simulink model "benchmark_model"  (R2021a)
settings: Solver=ode1  StartTime=0.0  StopTime=Tend  FixedStep=0.0001  MaxStep=0.1  MinStep=0.0001  AbsTol=0.01  EnableMultiTasking=on
undefined symbols (not defined in the file): A1, A2, AL, AM0, AREA, BORE, C_EGR, c_f, c_T, CAIR, cCO, cCO2, cH2, cH2O, cHC, cN2, CO, CO2, cO2, DEN0, DiscIntNeverNeededParam, EGR_dia, EGR_sk, EX_AREA, EX_M_AR, EXO, FD0, FOM, FR0, FR_C1, FR_C2, FR_C3, FR_C4, FR_C5, H2, H2O, HC, INC, INO, KET, Kex, Kh, MAS0, MCh, MHC, MN2, MO2, MOLcylT, N2, O2, PR0, R150, Rabs, SPEC, TBORE, Th_HC, Th_knock, THEX, THIN, TM0 ... (+9)
libraries: pid_lib x1
(part 6 of 6)

== matlab function benchmark_model/ENGINE/engine_s/cylinders/cyl2/cyl/Energy_Int/dvol/func_d_cylvol(u,SPEC)/Embedded MATLAB Function1 ==
  settings: fimath=|
      | fimath(...
      | 'RoundMode', 'floor',...
      | 'OverflowMode', 'wrap',...
      | 'ProductMode', 'KeepLSB', 'ProductWordLength', 32,...
      | 'SumMode', 'KeepLSB', 'SumWordLength', 32,...
      | 'CastBeforeSum', false)
  data: u input; y output; SPEC input size=19
function y = func_d_cylvol(u,SPEC)
%SPEC=[ 1:NCYL;  2:BORE;  3:STROKE;  4:RCRK;  5:CNTL;
%       6:COMP;  7:mc;    8:Jc;      9:cc;   10:mr;
%      11:Jr;   12:cr;   13:mp;     14:cp;   15:a;
%      16:b;    17:y_bdc;18:y_tdc;  19:Jfw;];

BORE   = SPEC(2);
STROKE = SPEC(3);
r      = SPEC(4);
l      = SPEC(5);
COMP   = SPEC(6);

AREA = 0.25*pi*BORE^2;
VH = AREA*STROKE;
VT = VH/(COMP-1);

LL = l^2-(r*sin(u))^2;
y = AREA*r*sin(u)*(1.0+r*cos(u)/sqrt(LL));

== matlab function benchmark_model/ENGINE/engine_s/cylinders/cyl1/ex_valve/cal_flow ==
  data: area input; fen output; inlet input; c_in input; outlet input; c_out input; fml output; WOM input
function [fen,fml] = func_nozzle(area,inlet,c_in,outlet,c_out,WOM) 
% made by Alex on February 3rd, 2010
% This program calculates the flow rate through the nozzle 
% under the assamption that the mass, the energy and the mometum
% are conserved between the inlet and the outlet flows.
%
% The inlet and the outlet are connected with the sign convention 
% of the calculated flow. The sign of the flow from th einlet and 
% the outlet is positive.
%
% inlet(1):pressure 
% inlet(2):density
% inlet(3):weight of molecule
% inlet(4):degree of freedom
% outlet(1):pressure 
% outlet(2):density
% outlet(3):weight of molecule
% outlet(4):degree of freedom

y = zeros(8,1); % modified 

du = inlet(1);
pu = inlet(2);
mu = inlet(3);
fu = inlet(4);
dd = outlet(1);
if dd<0
    dd=0;
end
pd = outlet(2);
md = outlet(3);
fd = outlet(4);
AR = area;

if (pu >= pd)
    rp = pd/pu;
    k = (fu + 2.0)/fu;
    crp = 1.0/(k + 1.0);
    A = AR*sqrt((k + 1.0)/(2.0*k)*abs(pu*du));
    B = sqrt((k/(k + 1.0))^2 - (0.99 - 1.0/(k + 1.0))^2);
    C = -(0.99 - 1.0/(k + 1.0))/B;
    a = (C*0.01 - B)/(2.0*0.01^3);
    c = C - 3.0*a*0.01^2;
    if (rp >= 0.99)
      fms = A*(a*(1.0 - rp)^3 + c*(1.0 - rp));
    else
      if (rp >= crp)
        R = (k/(k + 1.0))^2 - (rp - 1.0/(k + 1.0))^2;
        if (R < 0)
          R = 0;
        end
        fms = A*sqrt(R);
      else
        fms = A*k/(k + 1.0);
      end
    end
    fen = fms*(fu + 2.0)/2.0*pu/du;
    Ma = WOM'*c_in;
    fml = c_in*fms/Ma;
  else
    rp = pu/pd;
    k = (fd + 2.0)/fd;
    crp = 1.0/(k + 1.0);
    A = AR*sqrt((k + 1.0)/(2.0*k)*pd*dd);
    B = sqrt((k/(k + 1.0))^2 - (0.99 - 1.0/(k + 1.0))^2);
    C = (0.99 - 1.0/(k + 1.0))/B;
    a = (C*0.01 - B)/(2.0*0.01^3);
    c = C - 3.0*a*0.01^2;
    if (rp >= 0.99)
      fms = -A*(a*(1.0 - rp)^3 + c*(1.0 - rp));
    else
      if (rp >= crp)
        R = (k/(k + 1.0))^2 - (rp - 1.0/(k + 1.0))^2;
        if (R < 0)
          R = 0;
        end
        fms = -A*sqrt(R);
      else
        fms = -A*k/(k + 1.0);
      end
    end
    fen = fms*(fd + 2.0)/2.0*pd/dd;
    if isnan(fen)
        fen=0;
    end

    Ma = WOM'*c_out;
    fml = c_out*fms/Ma;
end
 if isnan(fen)||isinf(fen)
       fen=0;
end

== matlab function benchmark_model/ENGINE/engine_s/cylinders/cyl4/ex_valve/cal_flow ==
  data: area input; fen output; inlet input; c_in input; outlet input; c_out input; fml output; WOM input
function [fen,fml] = func_nozzle(area,inlet,c_in,outlet,c_out,WOM) 
% made by Alex on February 3rd, 2010
% This program calculates the flow rate through the nozzle 
% under the assamption that the mass, the energy and the mometum
% are conserved between the inlet and the outlet flows.
%
% The inlet and the outlet are connected with the sign convention 
% of the calculated flow. The sign of the flow from th einlet and 
% the outlet is positive.
%
% inlet(1):pressure 
% inlet(2):density
% inlet(3):weight of molecule
% inlet(4):degree of freedom
% outlet(1):pressure 
% outlet(2):density
% outlet(3):weight of molecule
% outlet(4):degree of freedom

y = zeros(8,1); % modified 

du = inlet(1);
pu = inlet(2);
mu = inlet(3);
fu = inlet(4);
dd = outlet(1);
if dd<0
    dd=0;
end
pd = outlet(2);
md = outlet(3);
fd = outlet(4);
AR = area;

if (pu >= pd)
    rp = pd/pu;
    k = (fu + 2.0)/fu;
    crp = 1.0/(k + 1.0);
    A = AR*sqrt((k + 1.0)/(2.0*k)*pu*du);
    B = sqrt((k/(k + 1.0))^2 - (0.99 - 1.0/(k + 1.0))^2);
    C = -(0.99 - 1.0/(k + 1.0))/B;
    a = (C*0.01 - B)/(2.0*0.01^3);
    c = C - 3.0*a*0.01^2;
    if (rp >= 0.99)
      fms = A*(a*(1.0 - rp)^3 + c*(1.0 - rp));
    else
      if (rp >= crp)
        R = (k/(k + 1.0))^2 - (rp - 1.0/(k + 1.0))^2;
        if (R < 0)
          R = 0;
        end
        fms = A*sqrt(R);
      else
        fms = A*k/(k + 1.0);
      end
    end
    fen = fms*(fu + 2.0)/2.0*pu/du;
    Ma = WOM'*c_in;
    fml = c_in*fms/Ma;
  else
    rp = pu/pd;
    k = (fd + 2.0)/fd;
    crp = 1.0/(k + 1.0);
    A = AR*sqrt((k + 1.0)/(2.0*k)*pd*dd);
    B = sqrt((k/(k + 1.0))^2 - (0.99 - 1.0/(k + 1.0))^2);
    C = (0.99 - 1.0/(k + 1.0))/B;
    a = (C*0.01 - B)/(2.0*0.01^3);
    c = C - 3.0*a*0.01^2;
    if (rp >= 0.99)
      fms = -A*(a*(1.0 - rp)^3 + c*(1.0 - rp));
    else
      if (rp >= crp)
        R = (k/(k + 1.0))^2 - (rp - 1.0/(k + 1.0))^2;
        if (R < 0)
          R = 0;
        end
        fms = -A*sqrt(R);
      else
        fms = -A*k/(k + 1.0);
      end
    end
    fen = fms*(fd + 2.0)/2.0*pd/dd;
    Ma = WOM'*c_out;
    fml = c_out*fms/Ma;
end
if isnan(fen)
       fen=0;
end

== matlab function benchmark_model/ENGINE/engine_s/cylinders/cyl4/in_valve/cal_flow ==
  data: area input; fen output; inlet input; c_in input; outlet input; c_out input; fml output; fms output; WOM input
function [fen,fml,fms] = func_nozzle(area,inlet,c_in,outlet,c_out,WOM) 
% made by Alex on February 3rd, 2010
% This program calculates the flow rate through the nozzle 
% under the assamption that the mass, the energy and the mometum
% are conserved between the inlet and the outlet flows.
%
% The inlet and the outlet are connected with the sign convention 
% of the calculated flow. The sign of the flow from th einlet and 
% the outlet is positive.
%
% inlet(1):pressure 
% inlet(2):density
% inlet(3):weight of molecule
% inlet(4):degree of freedom
% outlet(1):pressure 
% outlet(2):density
% outlet(3):weight of molecule
% outlet(4):degree of freedom

y = zeros(8,1); % modified 

du = inlet(1);
pu = inlet(2);
mu = inlet(3);
fu = inlet(4);
dd = outlet(1);
pd = outlet(2);
md = outlet(3);
fd = outlet(4);
AR = area;

if (pu >= pd)
    rp = pd/pu;
    k = (fu + 2.0)/fu;
    crp = 1.0/(k + 1.0);
    A = AR*sqrt((k + 1.0)/(2.0*k)*pu*du);
    B = sqrt((k/(k + 1.0))^2 - (0.99 - 1.0/(k + 1.0))^2);
    C = -(0.99 - 1.0/(k + 1.0))/B;
    a = (C*0.01 - B)/(2.0*0.01^3);
    c = C - 3.0*a*0.01^2;
    if (rp >= 0.99)
      fms = A*(a*(1.0 - rp)^3 + c*(1.0 - rp));
    else
      if (rp >= crp)
        R = (k/(k + 1.0))^2 - (rp - 1.0/(k + 1.0))^2;
        if (R < 0)
          R = 0;
        end
        fms = A*sqrt(R);
      else
        fms = A*k/(k + 1.0);
      end
    end
    fen = fms*(fu + 2.0)/2.0*pu/du;
    Ma = WOM'*c_in;
    fml = c_in*fms/Ma;
  else
    rp = pu/pd;
    k = (fd + 2.0)/fd;
    crp = 1.0/(k + 1.0);
    A = AR*sqrt((k + 1.0)/(2.0*k)*pd*dd);
    B = sqrt((k/(k + 1.0))^2 - (0.99 - 1.0/(k + 1.0))^2);
    C = (0.99 - 1.0/(k + 1.0))/B;
    a = (C*0.01 - B)/(2.0*0.01^3);
    c = C - 3.0*a*0.01^2;
    if (rp >= 0.99)
      fms = -A*(a*(1.0 - rp)^3 + c*(1.0 - rp));
    else
      if (rp >= crp)
        R = (k/(k + 1.0))^2 - (rp - 1.0/(k + 1.0))^2;
        if (R < 0)
          R = 0;
        end
        fms = -A*sqrt(R);
      else
        fms = -A*k/(k + 1.0);
      end
    end
    fen = fms*(fd + 2.0)/2.0*pd/dd;
    Ma = WOM'*c_out;
    fml = c_out*fms/Ma;
end
if isnan(fen)
    fen=0;
end

== matlab function benchmark_model/ENGINE/engine_s/cylinders/cyl1/in_valve/cal_flow ==
  data: area input; fen output; inlet input; c_in input; outlet input; c_out input; fml output; fms output; WOM input
function [fen,fml,fms] = func_nozzle(area,inlet,c_in,outlet,c_out,WOM) 
% made by Alex on February 3rd, 2010
% This program calculates the flow rate through the nozzle 
% under the assamption that the mass, the energy and the mometum
% are conserved between the inlet and the outlet flows.
%
% The inlet and the outlet are connected with the sign convention 
% of the calculated flow. The sign of the flow from th einlet and 
% the outlet is positive.
%
% inlet(1):pressure 
% inlet(2):density
% inlet(3):weight of molecule
% inlet(4):degree of freedom
% outlet(1):pressure 
% outlet(2):density
% outlet(3):weight of molecule
% outlet(4):degree of freedom

y = zeros(8,1); % modified 

du = inlet(1);
pu = inlet(2);
mu = inlet(3);
fu = inlet(4);
dd = outlet(1);
if dd<0
    dd=0;
end
pd = outlet(2);
md = outlet(3);
fd = outlet(4);
AR = area;

if (pu >= pd)
    rp = pd/pu;
    k = (fu + 2.0)/fu;
    crp = 1.0/(k + 1.0);
    A = AR*sqrt((k + 1.0)/(2.0*k)*pu*du);
    B = sqrt((k/(k + 1.0))^2 - (0.99 - 1.0/(k + 1.0))^2);
    C = -(0.99 - 1.0/(k + 1.0))/B;
    a = (C*0.01 - B)/(2.0*0.01^3);
    c = C - 3.0*a*0.01^2;
    if (rp >= 0.99)
      fms = A*(a*(1.0 - rp)^3 + c*(1.0 - rp));
    else
      if (rp >= crp)
        R = (k/(k + 1.0))^2 - (rp - 1.0/(k + 1.0))^2;
        if (R < 0)
          R = 0;
        end
        fms = A*sqrt(R);
      else
        fms = A*k/(k + 1.0);
      end
    end
    fen = fms*(fu + 2.0)/2.0*pu/du;
    Ma = WOM'*c_in;
    fml = c_in*fms/Ma;
  else
    rp = pu/pd;
    k = (fd + 2.0)/fd;
    crp = 1.0/(k + 1.0);
    A = AR*sqrt((k + 1.0)/(2.0*k)*pd*dd);
    B = sqrt((k/(k + 1.0))^2 - (0.99 - 1.0/(k + 1.0))^2);
    C = (0.99 - 1.0/(k + 1.0))/B;
    a = (C*0.01 - B)/(2.0*0.01^3);
    c = C - 3.0*a*0.01^2;
    if (rp >= 0.99)
      fms = -A*(a*(1.0 - rp)^3 + c*(1.0 - rp));
    else
      if (rp >= crp)
        R = (k/(k + 1.0))^2 - (rp - 1.0/(k + 1.0))^2;
        if (R < 0)
          R = 0;
        end
        fms = -A*sqrt(R);
      else
        fms = -A*k/(k + 1.0);
      end
    end
    fen = fms*(fd + 2.0)/2.0*pd/dd;
    Ma = WOM'*c_out;
    fml = c_out*fms/Ma;
end
if isnan(fen)
       fen=0;
end

== matlab function benchmark_model/ENGINE/engine_s/in_chamber/cal_flow ==
  data: area input; fen output; inlet input; c_in input; outlet input; c_out input; fml output; WOM input
function [fen,fml] = func_nozzle(area,inlet,c_in,outlet,c_out,WOM) 
% made by Alex on February 3rd, 2010
% This program calculates the flow rate through the nozzle 
% under the assamption that the mass, the energy and the mometum
% are conserved between the inlet and the outlet flows.
%
% The inlet and the outlet are connected with the sign convention 
% of the calculated flow. The sign of the flow from th einlet and 
% the outlet is positive.
%
% inlet(1):pressure 
% inlet(2):density
% inlet(3):weight of molecule
% inlet(4):degree of freedom
% outlet(1):pressure 
% outlet(2):density
% outlet(3):weight of molecule
% outlet(4):degree of freedom

y = zeros(8,1); % modified 

du = inlet(1);
pu = inlet(2);
mu = inlet(3);
fu = inlet(4);
dd = outlet(1);
pd = outlet(2);
md = outlet(3);
fd = outlet(4);
AR = area;

if (pu >= pd)
    rp = pd/pu;
    k = (fu + 2.0)/fu;
    crp = 1.0/(k + 1.0);
    A = AR*sqrt((k + 1.0)/(2.0*k)*pu*du);
    B = sqrt((k/(k + 1.0))^2 - (0.99 - 1.0/(k + 1.0))^2);
    C = -(0.99 - 1.0/(k + 1.0))/B;
    a = (C*0.01 - B)/(2.0*0.01^3);
    c = C - 3.0*a*0.01^2;
    if (rp >= 0.99)
      fms = A*(a*(1.0 - rp)^3 + c*(1.0 - rp));
    else
      if (rp >= crp)
        R = (k/(k + 1.0))^2 - (rp - 1.0/(k + 1.0))^2;
        if (R < 0)
          R = 0;
        end
        fms = A*sqrt(R);
      else
        fms = A*k/(k + 1.0);
      end
    end
    fen = fms*(fu + 2.0)/2.0*pu/du;
    Ma = WOM'*c_in;
    fml = c_in*fms/Ma;
  else
    rp = pu/pd;
    k = (fd + 2.0)/fd;
    crp = 1.0/(k + 1.0);
    A = AR*sqrt((k + 1.0)/(2.0*k)*pd*dd);
    B = sqrt((k/(k + 1.0))^2 - (0.99 - 1.0/(k + 1.0))^2);
    C = (0.99 - 1.0/(k + 1.0))/B;
    a = (C*0.01 - B)/(2.0*0.01^3);
    c = C - 3.0*a*0.01^2;
    if (rp >= 0.99)
      fms = -A*(a*(1.0 - rp)^3 + c*(1.0 - rp));
    else
      if (rp >= crp)
        R = (k/(k + 1.0))^2 - (rp - 1.0/(k + 1.0))^2;
        if (R < 0)
          R = 0;
        end
        fms = -A*sqrt(R);
      else
        fms = -A*k/(k + 1.0);
      end
    end
    fen = fms*(fd + 2.0)/2.0*pd/dd;
    Ma = WOM'*c_out;
    fml = c_out*fms/Ma;
end

== matlab function benchmark_model/ENGINE/engine_s/EGR_system/cal_flow ==
  data: area input; fen output; inlet input; c_in input; outlet input; c_out input; fml output; WOM input
function [fen,fml] = func_nozzle(area,inlet,c_in,outlet,c_out,WOM) 
% made by Alex on February 3rd, 2010
% This program calculates the flow rate through the nozzle 
% under the assamption that the mass, the energy and the mometum
% are conserved between the inlet and the outlet flows.
%
% The inlet and the outlet are connected with the sign convention 
% of the calculated flow. The sign of the flow from th einlet and 
% the outlet is positive.
%
% inlet(1):pressure 
% inlet(2):density
% inlet(3):weight of molecule
% inlet(4):degree of freedom
% outlet(1):pressure 
% outlet(2):density
% outlet(3):weight of molecule
% outlet(4):degree of freedom

y = zeros(8,1); % modified 
du = inlet(1);
if du<0
    du=0;
end
pu = inlet(2);
mu = inlet(3);
fu = inlet(4);
dd = outlet(1);
pd = outlet(2);
md = outlet(3);
fd = outlet(4);
AR = area;

if (pu >= pd)
    rp = pd/pu;
    k = (fu + 2.0)/fu;
    crp = 1.0/(k + 1.0);
    A = AR*sqrt((k + 1.0)/(2.0*k)*pu*du);
    B = sqrt((k/(k + 1.0))^2 - (0.99 - 1.0/(k + 1.0))^2);
    C = -(0.99 - 1.0/(k + 1.0))/B;
    a = (C*0.01 - B)/(2.0*0.01^3);
    c = C - 3.0*a*0.01^2;
    if (rp >= 0.99)
      fms = A*(a*(1.0 - rp)^3 + c*(1.0 - rp));
    else
      if (rp >= crp)
        R = (k/(k + 1.0))^2 - (rp - 1.0/(k + 1.0))^2;
        if (R < 0)
          R = 0;
        end
        fms = A*sqrt(R);
      else
        fms = A*k/(k + 1.0);
      end
    end
    fen = fms*(fu + 2.0)/2.0*pu/du;
    Ma = WOM'*c_in;
    fml = c_in*fms/Ma;
  else
    rp = pu/pd;
    k = (fd + 2.0)/fd;
    crp = 1.0/(k + 1.0);
    A = AR*sqrt((k + 1.0)/(2.0*k)*pd*dd);
    B = sqrt((k/(k + 1.0))^2 - (0.99 - 1.0/(k + 1.0))^2);
    C = (0.99 - 1.0/(k + 1.0))/B;
    a = (C*0.01 - B)/(2.0*0.01^3);
    c = C - 3.0*a*0.01^2;
    if (rp >= 0.99)
      fms = -A*(a*(1.0 - rp)^3 + c*(1.0 - rp));
    else
      if (rp >= crp)
        R = (k/(k + 1.0))^2 - (rp - 1.0/(k + 1.0))^2;
        if (R < 0)
          R = 0;
        end
        fms = -A*sqrt(R);
      else
        fms = -A*k/(k + 1.0);
      end
    end
    fen = fms*(fd + 2.0)/2.0*pd/dd;
    Ma = WOM'*c_out;
    fml = c_out*fms/Ma;
end
if isnan(fen)
       fen=0;
end

== matlab function benchmark_model/ENGINE/engine_s/cylinders/cyl2/cyl/cal_cyl_state/cyl_vol ==
  settings: fimath=|
      | fimath(...
      | 'RoundMode', 'floor',...
      | 'OverflowMode', 'wrap',...
      | 'ProductMode', 'KeepLSB', 'ProductWordLength', 32,...
      | 'SumMode', 'KeepLSB', 'SumWordLength', 32,...
      | 'CastBeforeSum', false)
  data: u input; vol output; SPEC input size=19
function vol=func_cylvol(u,SPEC)
%SPEC=[ 1:NCYL;  2:BORE;  3:STROKE;  4:RCRK;  5:CNTL;
%       6:COMP;  7:mc;    8:Jc;      9:cc;   10:mr;
%      11:Jr;   12:cr;   13:mp;     14:cp;   15:a;
%      16:b;    17:y_bdc;18:y_tdc;  19:Jfw;];

   r    = SPEC(4);
   l    = SPEC(5);
   
   AREA = 0.25*pi*SPEC(2)*SPEC(2);
   VH = AREA*SPEC(3);
   VT = VH/(SPEC(6)-1);
   LL = l^2-(r*sin(u))^2;
   vol = VT+AREA*((r+l)-(r*cos(u)+sqrt(LL)));

== matlab function benchmark_model/ENGINE/engine_s/cylinders/cyl2/cyl/frame/ratio_burnt1/murnt_ratio/Embedded MATLAB Function ==
  data: u input; q output; Web input; Q output
function [q,Q]  = func_webC_s(u,Web)
% made by Alex on January 28th, 2010
%   y: burnt ratio
%   u: crank angle that takes 0 at the compression TDC
% Web: parameters
%
WebA = Web(1);
WebM = Web(2);
WebT = Web(3);
WebS = Web(4);
WWebs = pi-WebS;

uu = mod(u,4*pi)-WWebs;
if (uu>0)   
    q = 1.0/WebT*(WebM+1.0)*WebA*(uu/WebT)^WebM*...
          exp(-WebA*(uu/WebT)^(WebM+1.0));
    Q = 1-exp(-WebA*(uu/WebT)^(WebM+1.0));
else
    q = 0;
    Q = 0;
end

== matlab function benchmark_model/ENGINE/engine_s/ex_chamber/cal_flow ==
  data: area input; fen output; inlet input; c_in input; outlet input; c_out input; fml output; WOM input
function [fen,fml] = func_nozzle(area,inlet,c_in,outlet,c_out,WOM) 
% made by Alex on February 3rd, 2010
% This program calculates the flow rate through the nozzle 
% under the assamption that the mass, the energy and the mometum
% are conserved between the inlet and the outlet flows.
%
% The inlet and the outlet are connected with the sign convention 
% of the calculated flow. The sign of the flow from th einlet and 
% the outlet is positive.
%
% inlet(1):pressure 
% inlet(2):density
% inlet(3):weight of molecule
% inlet(4):degree of freedom
% outlet(1):pressure 
% outlet(2):density
% outlet(3):weight of molecule
% outlet(4):degree of freedom

y = zeros(8,1); % modified 

du = inlet(1);
if du<0
    du=0;
end
pu = inlet(2);
mu = inlet(3);
fu = inlet(4);
dd = outlet(1);
pd = outlet(2);
md = outlet(3);
fd = outlet(4);
AR = area;

if (pu >= pd)
    rp = pd/pu;
    k = (fu + 2.0)/fu;
    crp = 1.0/(k + 1.0);
    A = AR*sqrt((k + 1.0)/(2.0*k)*pu*du);
    B = sqrt((k/(k + 1.0))^2 - (0.99 - 1.0/(k + 1.0))^2);
    C = -(0.99 - 1.0/(k + 1.0))/B;
    a = (C*0.01 - B)/(2.0*0.01^3);
    c = C - 3.0*a*0.01^2;
    if (rp >= 0.99)
      fms = A*(a*(1.0 - rp)^3 + c*(1.0 - rp));
    else
      if (rp >= crp)
        R = (k/(k + 1.0))^2 - (rp - 1.0/(k + 1.0))^2;
        if (R < 0)
          R = 0;
        end
        fms = A*sqrt(R);
      else
        fms = A*k/(k + 1.0);
      end
    end
    fen = fms*(fu + 2.0)/2.0*pu/du;
    Ma = WOM'*c_in;
    fml = c_in*fms/Ma;
  else
    rp = pu/pd;
    k = (fd + 2.0)/fd;
    crp = 1.0/(k + 1.0);
    A = AR*sqrt((k + 1.0)/(2.0*k)*pd*dd);
    B = sqrt((k/(k + 1.0))^2 - (0.99 - 1.0/(k + 1.0))^2);
    C = (0.99 - 1.0/(k + 1.0))/B;
    a = (C*0.01 - B)/(2.0*0.01^3);
    c = C - 3.0*a*0.01^2;
    if (rp >= 0.99)
      fms = -A*(a*(1.0 - rp)^3 + c*(1.0 - rp));
    else
      if (rp >= crp)
        R = (k/(k + 1.0))^2 - (rp - 1.0/(k + 1.0))^2;
        if (R < 0)
          R = 0;
        end
        fms = -A*sqrt(R);
      else
        fms = -A*k/(k + 1.0);
      end
    end
    fen = fms*(fd + 2.0)/2.0*pd/dd;
    Ma = WOM'*c_out;
    fml = c_out*fms/Ma;
end
if isnan(fen)
       fen=0;
end

== stateflow chart benchmark_model/ENGINE/engine_s/cylinders/cyl2/cyl/unburnt_gass/init&trig/qChart ==
  state A/
    exit:
    sl_out1=sl_in1;
    sl_out2=sl_in2;
    sl_out3=sl_in3;
    sl_out4=sl_in4;
    sl_out5=sl_in5;
    sl_out6=sl_in6;
    sl_out7=sl_in7;
  (default) -> A : {sl_out1=sl_in1;
      |  sl_out2=sl_in2;
      |  sl_out3=sl_in3;
      |  sl_out4=sl_in4;
      |  sl_out5=sl_in5;
      |  sl_out6=sl_in6;
      |  sl_out7=sl_in7;
      | }
  A -> A : event
  data: sl_in1 input; sl_out1 output double =NHC; sl_in2 input; sl_in3 input; sl_in4 input; sl_in5 input; sl_in6 input; sl_in7 input; sl_out2 output double =NCO2; sl_out3 output double =NCO; sl_out4 output double =NO2; sl_out5 output double =NH2; sl_out6 output double =NH2O; sl_out7 output double =NN2
  events: event input RISING_EDGE_EVENT

== matlab function benchmark_model/ENGINE/engine_s/cylinders/cyl2/ex_valve/cal_flow ==
  data: area input; fen output; inlet input; c_in input; outlet input; c_out input; fml output; WOM input
function [fen,fml] = func_nozzle(area,inlet,c_in,outlet,c_out,WOM) 
% made by Alex on February 3rd, 2010
% This program calculates the flow rate through the nozzle 
% under the assamption that the mass, the energy and the mometum
% are conserved between the inlet and the outlet flows.
%
% The inlet and the outlet are connected with the sign convention 
% of the calculated flow. The sign of the flow from th einlet and 
% the outlet is positive.
%
% inlet(1):pressure 
% inlet(2):density
% inlet(3):weight of molecule
% inlet(4):degree of freedom
% outlet(1):pressure 
% outlet(2):density
% outlet(3):weight of molecule
% outlet(4):degree of freedom

y = zeros(8,1); % modified 

du = inlet(1);
pu = inlet(2);
if pu<0
    pu=0;
end
mu = inlet(3);
fu = inlet(4);
dd = outlet(1);
if dd<0
    dd=0;
end
pd = outlet(2);
md = outlet(3);
fd = outlet(4);
AR = area;

if (pu >= pd)
    rp = pd/pu;
    k = (fu + 2.0)/fu;
    crp = 1.0/(k + 1.0);
    A = AR*sqrt((k + 1.0)/(2.0*k)*pu*du);
    B = sqrt((k/(k + 1.0))^2 - (0.99 - 1.0/(k + 1.0))^2);
    C = -(0.99 - 1.0/(k + 1.0))/B;
    a = (C*0.01 - B)/(2.0*0.01^3);
    c = C - 3.0*a*0.01^2;
    if (rp >= 0.99)
      fms = A*(a*(1.0 - rp)^3 + c*(1.0 - rp));
    else
      if (rp >= crp)
        R = (k/(k + 1.0))^2 - (rp - 1.0/(k + 1.0))^2;
        if (R < 0)
          R = 0;
        end
        fms = A*sqrt(R);
      else
        fms = A*k/(k + 1.0);
      end
    end
    fen = fms*(fu + 2.0)/2.0*pu/du;
    Ma = WOM'*c_in;
    fml = c_in*fms/Ma;
  else
    rp = pu/pd;
    k = (fd + 2.0)/fd;
    crp = 1.0/(k + 1.0);
    A = AR*sqrt((k + 1.0)/(2.0*k)*pd*dd);
    B = sqrt((k/(k + 1.0))^2 - (0.99 - 1.0/(k + 1.0))^2);
    C = (0.99 - 1.0/(k + 1.0))/B;
    a = (C*0.01 - B)/(2.0*0.01^3);
    c = C - 3.0*a*0.01^2;
    if (rp >= 0.99)
      fms = -A*(a*(1.0 - rp)^3 + c*(1.0 - rp));
    else
      if (rp >= crp)
        R = (k/(k + 1.0))^2 - (rp - 1.0/(k + 1.0))^2;
        if (R < 0)
          R = 0;
        end
        fms = -A*sqrt(R);
      else
        fms = -A*k/(k + 1.0);
      end
    end
    fen = fms*(fd + 2.0)/2.0*pd/dd;
    Ma = WOM'*c_out;
    fml = c_out*fms/Ma;
end
if isnan(fen)
       fen=0;
end

== matlab function benchmark_model/ENGINE/engine_s/cylinders/cyl2/in_valve/cal_flow ==
  data: area input; fen output; inlet input; c_in input; outlet input; c_out input; fml output; fms output; WOM input
function [fen,fml,fms] = func_nozzle(area,inlet,c_in,outlet,c_out,WOM) 
% made by Alex on February 3rd, 2010
% This program calculates the flow rate through the nozzle 
% under the assamption that the mass, the energy and the mometum
% are conserved between the inlet and the outlet flows.
%
% The inlet and the outlet are connected with the sign convention 
% of the calculated flow. The sign of the flow from th einlet and 
% the outlet is positive.
%
% inlet(1):pressure 
% inlet(2):density
% inlet(3):weight of molecule
% inlet(4):degree of freedom
% outlet(1):pressure 
% outlet(2):density
% outlet(3):weight of molecule
% outlet(4):degree of freedom

y = zeros(8,1); % modified 
du = inlet(1);
if du<0
    du=0;
end
pu = inlet(2);
mu = inlet(3);
fu = inlet(4);
dd = outlet(1);
if dd<0
    dd=1e-9;
end
pd = outlet(2);
md = outlet(3);
fd = outlet(4);
AR = area;

if (pu >= pd)
    rp = pd/pu;
    k = (fu + 2.0)/fu;
    crp = 1.0/(k + 1.0);
    A = AR*sqrt((k + 1.0)/(2.0*k)*pu*du);
    B = sqrt((k/(k + 1.0))^2 - (0.99 - 1.0/(k + 1.0))^2);
    C = -(0.99 - 1.0/(k + 1.0))/B;
    a = (C*0.01 - B)/(2.0*0.01^3);
    c = C - 3.0*a*0.01^2;
    if (rp >= 0.99)
      fms = A*(a*(1.0 - rp)^3 + c*(1.0 - rp));
    else
      if (rp >= crp)
        R = (k/(k + 1.0))^2 - (rp - 1.0/(k + 1.0))^2;
        if (R < 0)
          R = 0;
        end
        fms = A*sqrt(R);
      else
        fms = A*k/(k + 1.0);
      end
    end
    fen = fms*(fu + 2.0)/2.0*pu/du;
    Ma = WOM'*c_in;
    fml = c_in*fms/Ma;
  else
    rp = pu/pd;
    k = (fd + 2.0)/fd;
    crp = 1.0/(k + 1.0);
    A = AR*sqrt((k + 1.0)/(2.0*k)*pd*dd);
    B = sqrt((k/(k + 1.0))^2 - (0.99 - 1.0/(k + 1.0))^2);
    C = (0.99 - 1.0/(k + 1.0))/B;
    a = (C*0.01 - B)/(2.0*0.01^3);
    c = C - 3.0*a*0.01^2;
    if (rp >= 0.99)
      fms = -A*(a*(1.0 - rp)^3 + c*(1.0 - rp));
    else
      if (rp >= crp)
        R = (k/(k + 1.0))^2 - (rp - 1.0/(k + 1.0))^2;
        if (R < 0)
          R = 0;
        end
        fms = -A*sqrt(R);
      else
        fms = -A*k/(k + 1.0);
      end
    end
    fen = fms*(fd + 2.0)/2.0*pd/dd;
    Ma = WOM'*c_out;
    fml = c_out*fms/Ma;
end
 if isnan(fen)
       fen=0;
end
